simulink model "P Controller"  (R2021a)
settings: Solver=VariableStepAuto  StartTime=0.0  StopTime=10  MaxStep=0.01  RelTol=1e-3
settings Model: Creator=haden  LastModifiedBy=haden

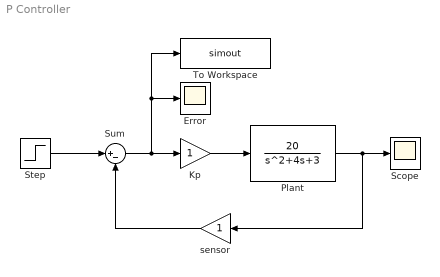
== system P Controller ==
  Error : Scope
  Kp : Gain
  Plant : TransferFcn  Numerator=[20]  Denominator=[1 4 3]
  Scope : Scope
  Step : Step  SampleTime=0
  Sum : Sum  Inputs=|+-
  To Workspace : ToWorkspace  VariableName=simout  SaveFormat=Structure With Time  SampleTime=-1
  sensor : Gain
  wires:
  Plant/1 -> sensor/1, Scope/1
  Kp/1 -> Plant/1
  Step/1 -> Sum/1
  Sum/1 -> To Workspace/1, Error/1, Kp/1
  sensor/1 -> Sum/2
